simulink model "OR_AND_XOR"  (R2023b)
settings: Solver=VariableStepAuto  StartTime=0.0  StopTime=10.0  RelTol=1e-3
settings Model: Creator=egzaragosin  LastModifiedBy=egzaragosin

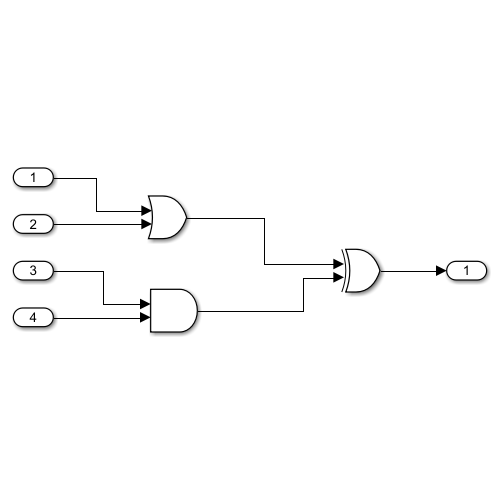
[thumbnail: Simulink's stored preview of the top-level diagram]
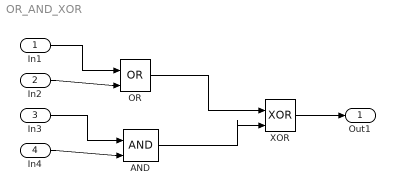
== system OR_AND_XOR ==
  In1 : Inport  OutDataTypeStr=boolean
  In2 : Inport  Port=2  OutDataTypeStr=boolean
  In3 : Inport  Port=3  OutDataTypeStr=boolean
  In4 : Inport  Port=4  OutDataTypeStr=boolean
  AND : Logic  IconShape=distinctive  AllPortsSameDT=off  OutDataTypeStr=boolean
  OR : Logic  Operator=OR  IconShape=distinctive  AllPortsSameDT=off  OutDataTypeStr=boolean
  XOR : Logic  Operator=XOR  IconShape=distinctive  AllPortsSameDT=off  OutDataTypeStr=boolean
  Out1 : Outport  OutDataTypeStr=boolean
  wires:
  OR/1 -> XOR/1
  AND/1 -> XOR/2
  In1/1 -> OR/1
  In2/1 -> OR/2
  In3/1 -> AND/1
  In4/1 -> AND/2
  XOR/1 -> Out1/1
